simulink model "dc_mot_transient_ideal_voltage_without_controller"  (R2019b)
settings: Solver=VariableStepAuto  StartTime=0.0  StopTime=1  RelTol=1e-3
settings Model: Creator=srikesh  LastModifiedBy=srikesh

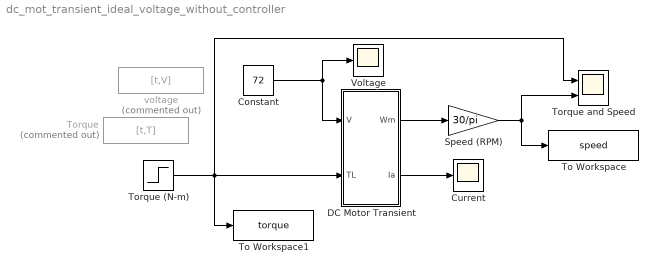
== system dc_mot_transient_ideal_voltage_without_controller ==
  Constant : Constant  Value=72
  Current : Scope
  "DC Motor Transient " : Subsystem  mask{Ra=.1472, Ke=1.27, Kt=.9852, J=.01, b=.005}
      mask prompts: Ra "Ra(Ohm)"; Ke "Ke(V-s)"; Kt "Kt(N-m/A)"; J "J(kg-m^2)"; b "b(N-m-s)"
  "Speed (RPM) " : Gain  Gain=30/pi
  To Workspace : ToWorkspace  VariableName=speed  SaveFormat=Timeseries  SampleTime=-1
  To Workspace1 : ToWorkspace  VariableName=torque  SaveFormat=Timeseries  SampleTime=-1
  "Torque " : FromWorkspace  Commented=on  VariableName=[t,T]  SampleTime=0
  Torque (N-m) : Step  Time=0  After=20  SampleTime=0
  Torque and Speed : Scope  NumInputPorts=2
  Voltage : Scope
  voltage : FromWorkspace  Commented=on  VariableName=[t,V]  SampleTime=0
  wires:
  Torque (N-m)/1 -> Torque and Speed/1, "DC Motor Transient "/2("TL "), To Workspace1/1
  "DC Motor Transient "/2(Ia) -> Current/1
  Constant/1 -> "DC Motor Transient "/1("V "), Voltage/1
  "DC Motor Transient "/1("Wm ") -> "Speed (RPM) "/1
  "Speed (RPM) "/1 -> To Workspace/1, Torque and Speed/2

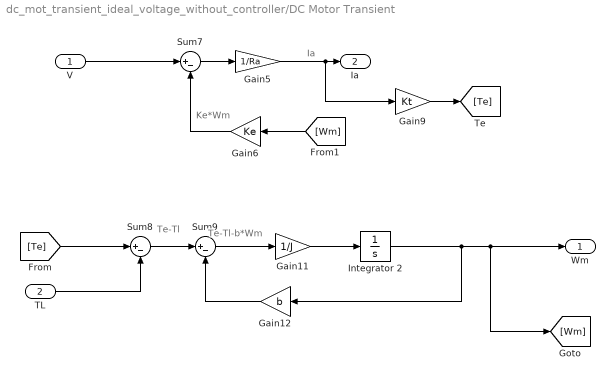
== system dc_mot_transient_ideal_voltage_without_controller/DC Motor Transient  ==
  note: Te-Tl-b*Wm
  note: Te-Tl
  note: Ia
  note: Ke*Wm
  "V " : Inport
  "TL " : Inport  Port=2
  Gain11 : Gain  Gain=1/J
  Gain12 : Gain  Gain=b
  Gain5 : Gain  Gain=1/Ra
  Gain6 : Gain  Gain=Ke
  Gain9 : Gain  Gain=Kt
  Integrator 2 : Integrator
  Sum7 : Sum  Inputs=|+-
  Sum8 : Sum  Inputs=|+-
  Sum9 : Sum  Inputs=|+-
  "Wm " : Outport
  Ia : Outport  Port=2
  wires:
  "V "/1 -> Sum7/1
  Gain6/1 -> Sum7/2
  Gain12/1 -> Sum9/2
  [Te] -> Sum8/1
  [Wm] -> Gain6/1
  Sum8/1 -> Sum9/1
  Gain9/1 -> [Te]
  "TL "/1 -> Sum8/2
  Gain11/1 -> Integrator 2/1
  Sum9/1 -> Gain11/1
  Integrator 2/1 -> Gain12/1, "Wm "/1, [Wm]
  Sum7/1 -> Gain5/1
  Gain5/1 -> Gain9/1, Ia/1
